simulink model "foc_closed_loop_test"  (R2015a)
settings: Solver=ode45  StartTime=0.0  StopTime=2  RelTol=1e-3
libraries: simulink x2
settings Model: Creator=user  LastModifiedBy=user

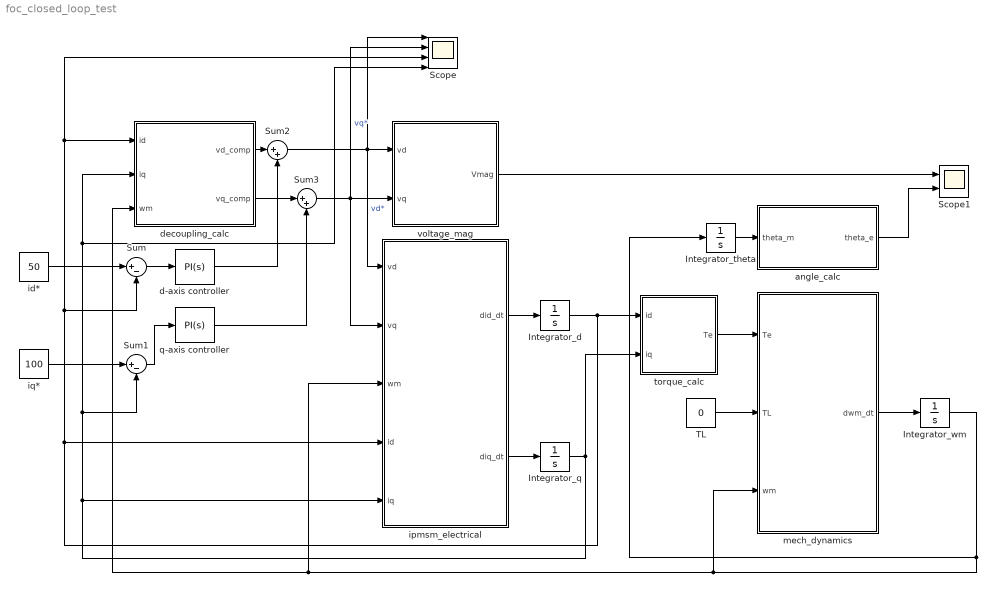
== system foc_closed_loop_test ==
  Integrator_d : Integrator
  Integrator_q : Integrator
  Integrator_theta : Integrator
  Integrator_wm : Integrator
  Scope : Scope  NumInputPorts=4
      settings: YMin=-5~-5~-5~-5  YMax=5~5~5~5  SaveName=ScopeData2
  Scope1 : Scope  NumInputPorts=2
      settings: YMin=-5~-5  YMax=5~5
  Sum : Sum  Inputs=|+-
  Sum1 : Sum  Inputs=|+-
  Sum2 : Sum  Inputs=|++
  Sum3 : Sum  Inputs=|++
  TL : Constant  Value=0
  angle_calc : MATLAB Function  TreatAsAtomicUnit=on
  d-axis controller : simulink/Continuous/PID Controller  Controller=PI  TimeDomain=Continuous-time  SampleTime=-1  IntegratorMethod=Forward Euler  FilterMethod=Forward Euler  Form=Parallel  UseFilter=on  ControllerParametersSource=internal  P=0.2827  I=16.6504  D=0  N=100  InitialConditionSource=internal  InitialConditionForIntegrator=0  InitialConditionForFilter=0  ExternalReset=none  LimitOutput=off  UpperSaturationLimit=inf  LowerSaturationLimit=-inf  LinearizeAsGain=on  AntiWindupMode=none  Kb=1  TrackingMode=off  Kt=1  PParamMin=[]  PParamMax=[]  IParamMin=[]  IParamMax=[]  DParamMin=[]  DParamMax=[]  NParamMin=[]  NParamMax=[]  KbParamMin=[]  KbParamMax=[]  KtParamMin=[]  KtParamMax=[]  POutMin=[]  POutMax=[]  IOutMin=[]  IOutMax=[]  DOutMin=[]  DOutMax=[]  NOutMin=[]  NOutMax=[]  KbOutMin=[]  KbOutMax=[]  KtOutMin=[]  KtOutMax=[]  IntegratorOutMin=[]  IntegratorOutMax=[]  FilterOutMin=[]  FilterOutMax=[]  SumOutMin=[]  SumOutMax=[]  SumI1OutMin=[]  SumI1OutMax=[]  SumI2OutMin=[]  SumI2OutMax=[]  SumI3OutMin=[]  SumI3OutMax=[]  SumDOutMin=[]  SumDOutMax=[]  SaturationOutMin=[]  SaturationOutMax=[]  IntegratorContinuousStateAttributes=''  IntegratorStateMustResolveToSignalObject=off  IntegratorRTWStateStorageClass=Auto  FilterContinuousStateAttributes=''  FilterStateMustResolveToSignalObject=off  FilterRTWStateStorageClass=Auto  DifferentiatorICPrevScaledInput=0  DifferentiatorOutMin=[]  DifferentiatorOutMax=[]
  decoupling_calc : MATLAB Function  TreatAsAtomicUnit=on
  id* : Constant  Value=50
  ipmsm_electrical : MATLAB Function  TreatAsAtomicUnit=on
  iq* : Constant  Value=100
  mech_dynamics : MATLAB Function  TreatAsAtomicUnit=on
  q-axis controller : simulink/Continuous/PID Controller  Controller=PI  TimeDomain=Continuous-time  SampleTime=-1  IntegratorMethod=Forward Euler  FilterMethod=Forward Euler  Form=Parallel  UseFilter=on  ControllerParametersSource=internal  P=0.8011  I=16.6504  D=0  N=100  InitialConditionSource=internal  InitialConditionForIntegrator=0  InitialConditionForFilter=0  ExternalReset=none  LimitOutput=off  UpperSaturationLimit=inf  LowerSaturationLimit=-inf  LinearizeAsGain=on  AntiWindupMode=none  Kb=1  TrackingMode=off  Kt=1  PParamMin=[]  PParamMax=[]  IParamMin=[]  IParamMax=[]  DParamMin=[]  DParamMax=[]  NParamMin=[]  NParamMax=[]  KbParamMin=[]  KbParamMax=[]  KtParamMin=[]  KtParamMax=[]  POutMin=[]  POutMax=[]  IOutMin=[]  IOutMax=[]  DOutMin=[]  DOutMax=[]  NOutMin=[]  NOutMax=[]  KbOutMin=[]  KbOutMax=[]  KtOutMin=[]  KtOutMax=[]  IntegratorOutMin=[]  IntegratorOutMax=[]  FilterOutMin=[]  FilterOutMax=[]  SumOutMin=[]  SumOutMax=[]  SumI1OutMin=[]  SumI1OutMax=[]  SumI2OutMin=[]  SumI2OutMax=[]  SumI3OutMin=[]  SumI3OutMax=[]  SumDOutMin=[]  SumDOutMax=[]  SaturationOutMin=[]  SaturationOutMax=[]  IntegratorContinuousStateAttributes=''  IntegratorStateMustResolveToSignalObject=off  IntegratorRTWStateStorageClass=Auto  FilterContinuousStateAttributes=''  FilterStateMustResolveToSignalObject=off  FilterRTWStateStorageClass=Auto  DifferentiatorICPrevScaledInput=0  DifferentiatorOutMin=[]  DifferentiatorOutMax=[]
  torque_calc : MATLAB Function  TreatAsAtomicUnit=on
  voltage_mag : MATLAB Function  TreatAsAtomicUnit=on
  wires:
  id*/1 -> Sum/1
  Sum/1 -> d-axis controller/1
  iq*/1 -> Sum1/1
  Integrator_q/1 -> decoupling_calc/2(iq), Scope/4, Sum1/2, ipmsm_electrical/5(iq), torque_calc/2(iq)
  Sum1/1 -> q-axis controller/1
  ipmsm_electrical/2(diq_dt) -> Integrator_q/1
  ipmsm_electrical/1(did_dt) -> Integrator_d/1
  Integrator_d/1 -> torque_calc/1(id), Scope/3, decoupling_calc/1(id), Sum/2, ipmsm_electrical/4(id)
  Integrator_wm/1 -> Integrator_theta/1, mech_dynamics/3(wm), ipmsm_electrical/3(wm), decoupling_calc/3(wm)
  decoupling_calc/1(vd_comp) -> Sum2/1
  d-axis controller/1 -> Sum2/2
  decoupling_calc/2(vq_comp) -> Sum3/1
  q-axis controller/1 -> Sum3/2
  Sum3/1 -> Scope/2, voltage_mag/2(vq), ipmsm_electrical/2(vq)  "vq*"
  Sum2/1 -> ipmsm_electrical/1(vd), voltage_mag/1(vd), Scope/1  "vd*"
  torque_calc/1(Te) -> mech_dynamics/1(Te)
  TL/1 -> mech_dynamics/2(TL)
  mech_dynamics/1(dwm_dt) -> Integrator_wm/1
  Integrator_theta/1 -> angle_calc/1(theta_m)
  voltage_mag/1(Vmag) -> Scope1/1
  angle_calc/1(theta_e) -> Scope1/2

== matlab function foc_closed_loop_test/decoupling_calc ==
  data: id input; vd_comp output; iq input; wm input; vq_comp output
function [vd_comp, vq_comp] = decoupling_calc(id, iq, wm)
% Feedforward decoupling terms for BMW i3 IPMSM

Ld       = 0.090e-3;
Lq       = 0.255e-3;
lambda_m = 0.0385;
p        = 6;

we = p*wm;

vd_comp = -we*Lq*iq;
vq_comp =  we*(Ld*id + lambda_m);

end

== matlab function foc_closed_loop_test/ipmsm_electrical ==
  data: vd input; did_dt output; vq input; wm input; id input; iq input; diq_dt output
function [did_dt, diq_dt] = ipmsm_electrical(vd, vq, wm, id, iq)
% BMW i3 IPMSM dq-axis electrical dynamics
% Units: V, rad/s, A, A/s

Rs       = 5.3e-3;    % Stator resistance, Ohm
Ld       = 0.090e-3;  % d-axis inductance, H
Lq       = 0.255e-3;  % q-axis inductance, H
lambda_m = 0.0385;    % PM flux linkage, Wb
p        = 6;         % Pole pairs

we = p*wm;             % electrical angular velocity, rad/s

did_dt = (vd - Rs*id + we*Lq*iq) / Ld;
diq_dt = (vq - Rs*iq - we*(Ld*id + lambda_m)) / Lq;

end

== matlab function foc_closed_loop_test/torque_calc ==
  data: id input; Te output; iq input
function Te = torque_calc(id, iq)
% BMW i3 electromagnetic torque
% Units: id, iq in A; Te in Nm

Ld       = 0.090e-3;
Lq       = 0.255e-3;
lambda_m = 0.0385;
p        = 6;

Te = (3/2) * p * (lambda_m*iq + (Ld - Lq)*id*iq);

end

== matlab function foc_closed_loop_test/mech_dynamics ==
  data: Te input; dwm_dt output; TL input; wm input
function dwm_dt = mech_dynamics(Te, TL, wm)
% BMW i3 mechanical dynamics
% Units: Te, TL in Nm; wm in rad/s; dwm_dt in rad/s^2

J = 0.06;    % ASSUMED
B = 0.001;   % ASSUMED

dwm_dt = (Te - TL - B*wm) / J;

end

== matlab function foc_closed_loop_test/angle_calc ==
  data: theta_m input; theta_e output
function theta_e = angle_calc(theta_m)
% Electrical angle from mechanical angle
p = 6;
theta_e = p*theta_m;
end

== matlab function foc_closed_loop_test/voltage_mag ==
  data: vd input; Vmag output; vq input
function Vmag = voltage_mag(vd, vq)
% Commanded voltage vector magnitude
Vmag = sqrt(vd^2 + vq^2);
end
